simulink model "DiscreteIntegrator_TestGen3"  (R2017b)
settings: Solver=FixedStepDiscrete  StartTime=0.0  StopTime=10.0  RelTol=1e-3
undefined symbols (not defined in the file): Block_TestLib, DiscIntNeverNeededParam, reset
settings Model: Creator=hbourbou  LastModifiedBy=hbourbou
settings DebuggingCC: ParameterOverflowMsg=none

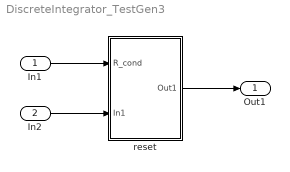
== system DiscreteIntegrator_TestGen3 ==
  In1 : Inport
  In2 : Inport  Port=2
  reset : Subsystem  AncestorBlock=Block_TestLib/reset
  Out1 : Outport
  wires:
  In1/1 -> reset/1(R_cond)
  In2/1 -> reset/2(In1)
  reset/1(Out1) -> Out1/1

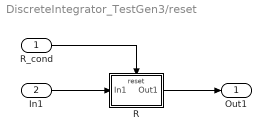
== system DiscreteIntegrator_TestGen3/reset ==
  R_cond : Inport  OutDataTypeStr=boolean
  In1 : Inport  Port=2
  R : Subsystem  TreatAsAtomicUnit=on
  Out1 : Outport
  wires:
  R_cond/1 -> R/Reset
  In1/1 -> R/1(In1)
  R/1(Out1) -> Out1/1

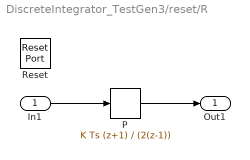
== system DiscreteIntegrator_TestGen3/reset/R ==
  In1 : Inport  PortDimensions=2
  Reset : ResetPort  DisableCoverage=on
  P : DiscreteIntegrator  IntegratorMethod=Integration: Trapezoidal  InitialCondition=7  InitialConditionSetting=State (most efficient)  SampleTime=-1  OutDataTypeStr=double  UpperSaturationLimit=100  LowerSaturationLimit=5  ICPrevOutput=DiscIntNeverNeededParam  ICPrevScaledInput=DiscIntNeverNeededParam
  Out1 : Outport
  wires:
  In1/1 -> P/1
  P/1 -> Out1/1
